simulink model "model"  (R2022a)
settings: Solver=ode113  StartTime=0  StopTime=1.5  MaxStep=1e-3
values from neighbouring files (symbols this model uses):
  argD = [1 -2 1 0 0]    [solves.m]
  argU = [k 2*(k+3) -4*(k+3) 2*(k+3)]    [solves.m]
  currentmodel = 5    [solves.m]
  eqSolve = eq5Solve    [solves.m]
  InputGt2 = 0    [solves.m]
  k = 7 + 1    (= 8)    [solves.m]
libraries: simulink x3
settings Model: Creator=Administrator  LastModifiedBy=Administrator
settings SolverCC: MaxConsecutiveMinStep=1000  ZeroCrossAlgorithm=Adaptive  ODENIntegrationMethod=ode4

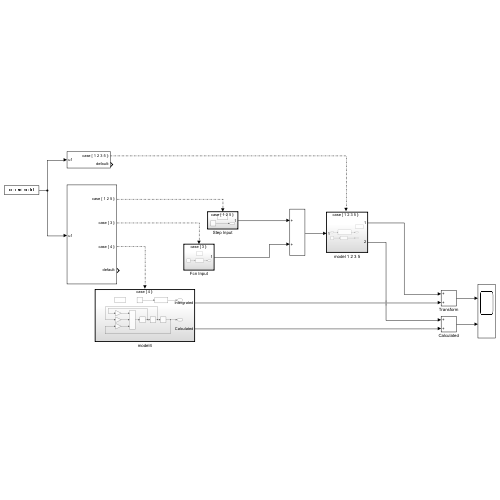
[thumbnail: Simulink's stored preview of the top-level diagram]
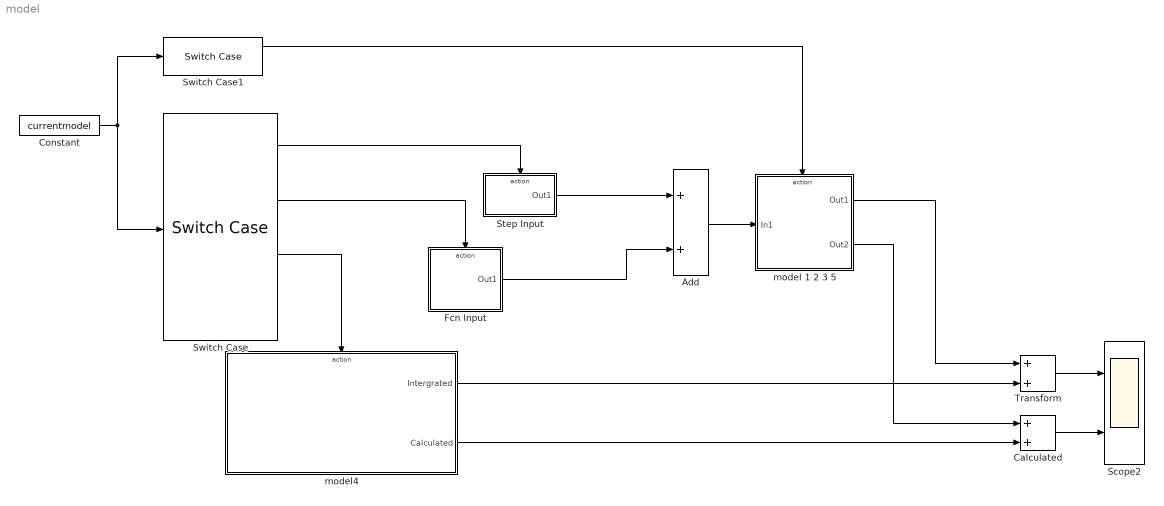
== system model ==
  Add : Sum
  Calculated : Sum
  Constant : Constant  Value=currentmodel
  Fcn Input : Subsystem
  Scope2 : Scope  NumInputPorts=2
  Step Input : Subsystem
  Switch Case : SwitchCase  CaseConditions={[1,2,5],3,4}
  Switch Case1 : SwitchCase  CaseConditions={[1,2,3,5]}
  Transform : Sum
  model 1 2 3 5 : Subsystem
  model4 : Subsystem
  wires:
  Add/1 -> model 1 2 3 5/1(In1)
  Constant/1 -> Switch Case/1, Switch Case1/1
  Transform/1 -> Scope2/1
  Calculated/1 -> Scope2/2
  model4/1(Intergrated) -> Transform/2
  model4/2(Calculated) -> Calculated/2
  Switch Case/3 -> model4/Action
  Fcn Input/1(Out1) -> Add/2
  Switch Case/1 -> Step Input/Action
  Switch Case/2 -> Fcn Input/Action
  Step Input/1(Out1) -> Add/1
  model 1 2 3 5/1(Out1) -> Transform/1
  model 1 2 3 5/2(Out2) -> Calculated/1
  Switch Case1/1 -> model 1 2 3 5/Action

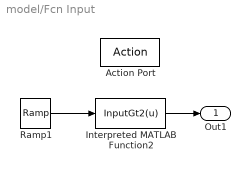
== system model/Fcn Input ==
  Action Port : ActionPort  ActionPortLabel=case [ 3 ]:
  Interpreted MATLAB Function2 : MATLABFcn  MATLABFcn=InputGt2(u)
  Ramp1 : simulink/Sources/Ramp  slope=1  start=0  InitialOutput=0
  Out1 : Outport
  wires:
  Interpreted MATLAB Function2/1 -> Out1/1
  Ramp1/1 -> Interpreted MATLAB Function2/1

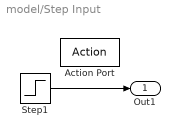
== system model/Step Input ==
  Action Port : ActionPort  ActionPortLabel=case [ 1 2 5 ]:
  Step1 : Step  Time=0  SampleTime=0
  Out1 : Outport
  wires:
  Step1/1 -> Out1/1

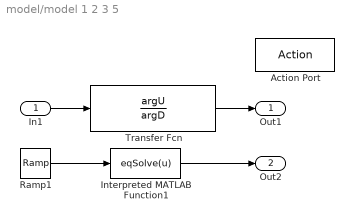
== system model/model 1 2 3 5 ==
  In1 : Inport
  Action Port : ActionPort  ActionPortLabel=case [ 1 2 3 5 ]:
  Interpreted MATLAB Function1 : MATLABFcn  MATLABFcn=eqSolve(u)
  Ramp1 : simulink/Sources/Ramp  slope=1  start=0  InitialOutput=0
  Transfer Fcn : TransferFcn  Numerator=argU  Denominator=argD
  Out1 : Outport
  Out2 : Outport  Port=2
  wires:
  In1/1 -> Transfer Fcn/1
  Transfer Fcn/1 -> Out1/1
  Interpreted MATLAB Function1/1 -> Out2/1
  Ramp1/1 -> Interpreted MATLAB Function1/1

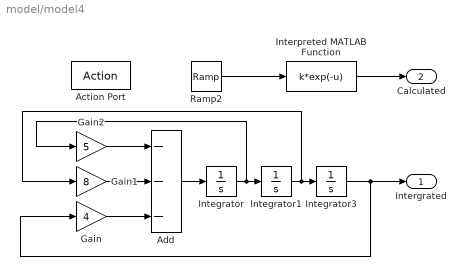
== system model/model4 ==
  Action Port : ActionPort  ActionPortLabel=case [ 4 ]:
  Add : Sum  Inputs=---
  Gain : Gain  Gain=4
  Gain1 : Gain  Gain=8
  Gain2 : Gain  Gain=5
  Integrator : Integrator  InitialCondition=k
  Integrator1 : Integrator  InitialCondition=-k
  Integrator3 : Integrator  InitialCondition=k
  Interpreted MATLAB Function : MATLABFcn  MATLABFcn=k*exp(-u)
  Ramp2 : simulink/Sources/Ramp  slope=1  start=0  InitialOutput=0
  Intergrated : Outport
  Calculated : Outport  Port=2
  wires:
  Interpreted MATLAB Function/1 -> Calculated/1
  Integrator1/1 -> Gain1/1, Integrator3/1
  Gain2/1 -> Add/1
  Add/1 -> Integrator/1
  Ramp2/1 -> Interpreted MATLAB Function/1
  Gain/1 -> Add/3
  Integrator3/1 -> Gain/1, Intergrated/1
  Gain1/1 -> Add/2
  Integrator/1 -> Gain2/1, Integrator1/1
